simulink model "AGTF30SysDyn_PExPIn"  (R2023b)
settings: Solver=ode4  StartTime=0.0  StopTime=MWS.In.tend  FixedStep=MWS.In.Ts  RelTol=1e-3  EnableMultiTasking=on
model workspace: external: MAT-File (data not in the file)
values from neighbouring files (symbols this model uses):
  MWS = setup_initialize(MWS,startPt,SSsolverSP)    [Setup_Simulation.m]    (also in run_AGTF30e_script.m = Setup_Simulation(inputMethod,MWS.In,filename,Mdl,SSsolverSP))
undefined symbols (not defined in the file or in its folder): DiscIntNeverNeededParam
libraries: simulink x32, Lib_Solve_ModelSource_TMATS x28, Lib_EMTAT x27, Lib_Cntrl_FirstOrderSensor_TMATS x19, Lib_Cntrl_FirstOrderActuator_TMATS x2, Lib_Cntrl_LimitSelect_TMATS x2, Lib_Solve_OuterLoopIntegrator_TMATS x2, Lib_Cntrl_CorrectedSpeed_TMATS x1, Lib_Solve_IterNRSolverJC_TMATS x1, slpidlib x1
(part 3 of 8)

== system AGTF30SysDyn_PExPIn/Control System/Electric Machine Controllers/TEEM Power ==
  k_N1cErrN : Inport
  f_N1cErrN : Inport  Port=2
  Prelookup : Inport  Port=3
  Bus Selector1 : BusSelector  OutputSignals=k_Alt,f_Alt
  Constant : Constant  Value=MWS.In.Options.TEEM
  Constant1 : Constant  Value=0
  PwrExAccel Interpolation Using Prelookup : Interpolation_n-D  Table=MWS.Cntrl.TEEM.PwrExAccel.Pwr_array  InternalRulePriority=Speed
  PwrInAccel Interpolation Using Prelookup : Interpolation_n-D  Table=MWS.Cntrl.TEEM.PwrInAccel.Pwr_array  InternalRulePriority=Speed
  PwrXDecel Interpolation Using Prelookup : Interpolation_n-D  Table=MWS.Cntrl.TEEM.PwrXDecel.Pwr_array  InternalRulePriority=Speed
  Switch : Switch  Criteria=u2 > Threshold  SaturateOnIntegerOverflow=off  InputSameDT=off
  Switch1 : Switch  Criteria=u2 > Threshold  SaturateOnIntegerOverflow=off  InputSameDT=off
  Switch2 : Switch  Criteria=u2 > Threshold  SaturateOnIntegerOverflow=off  InputSameDT=off
  PwrInAccel_TEEM : Outport
  PwrExAccel_TEEM : Outport  Port=2
  PwrXDecel_TEEM : Outport  Port=3
  wires:
  Prelookup/1 -> Bus Selector1/1
  PwrInAccel Interpolation Using Prelookup/1 -> Switch/1  "PwrInAccel_TEEM"
  Bus Selector1/2 -> PwrExAccel Interpolation Using Prelookup/4, PwrInAccel Interpolation Using Prelookup/4, PwrXDecel Interpolation Using Prelookup/4  "<f_Alt>"
  k_N1cErrN/1 -> PwrExAccel Interpolation Using Prelookup/1, PwrInAccel Interpolation Using Prelookup/1, PwrXDecel Interpolation Using Prelookup/1
  PwrXDecel Interpolation Using Prelookup/1 -> Switch1/1  "PwrXDecel_TEEM"
  f_N1cErrN/1 -> PwrExAccel Interpolation Using Prelookup/2, PwrInAccel Interpolation Using Prelookup/2, PwrXDecel Interpolation Using Prelookup/2
  Bus Selector1/1 -> PwrExAccel Interpolation Using Prelookup/3, PwrInAccel Interpolation Using Prelookup/3, PwrXDecel Interpolation Using Prelookup/3  "<k_Alt>"
  Constant/1 -> Switch2/2, Switch1/2, Switch/2
  Switch/1 -> PwrInAccel_TEEM/1
  Switch1/1 -> PwrXDecel_TEEM/1
  PwrExAccel Interpolation Using Prelookup/1 -> Switch2/1  "PwrExAccel_TEEM"
  Constant1/1 -> Switch1/3, Switch2/3, Switch/3
  Switch2/1 -> PwrExAccel_TEEM/1

== system AGTF30SysDyn_PExPIn/Control System/Scheduling/MaxMin Fuel Flow Calc ==
  k_Alt : Inport
  f_Alt : Inport  Port=2
  k_MN : Inport  Port=3
  f_MN : Inport  Port=4
  k_PwrInLPMx : Inport  Port=5
  f_PwrInLPMx : Inport  Port=6
  k_PwrInLPMn : Inport  Port=7
  f_PwrInLPMn : Inport  Port=8
  k_PwrInHPMx : Inport  Port=9
  f_PwrInHPMx : Inport  Port=10
  k_PwrInHPMn : Inport  Port=11
  f_PwrInHPMn : Inport  Port=12
  Wfmax Interpolation Using Prelookup : Interpolation_n-D  NumberOfTableDimensions=4  Table=MWS.Cntrl.Sched.WfMax.WfMax_array  InternalRulePriority=Speed
      settings: InputPortMap=u0,u1,u2,u3,u4,u5,u6,u7
  Wfmin Interpolation Using Prelookup : Interpolation_n-D  NumberOfTableDimensions=4  Table=MWS.Cntrl.Sched.WfMin.WfMin_array  InternalRulePriority=Speed
      settings: InputPortMap=u0,u1,u2,u3,u4,u5,u6,u7
  Wfmin : Outport  VectorParamsAs1DForOutWhenUnconnected=off
  Wfmax : Outport  Port=2  VectorParamsAs1DForOutWhenUnconnected=off
  wires:
  f_PwrInLPMn/1 -> Wfmin Interpolation Using Prelookup/6
  k_PwrInLPMn/1 -> Wfmin Interpolation Using Prelookup/5
  f_PwrInLPMx/1 -> Wfmax Interpolation Using Prelookup/6
  k_PwrInLPMx/1 -> Wfmax Interpolation Using Prelookup/5
  f_MN/1 -> Wfmax Interpolation Using Prelookup/4, Wfmin Interpolation Using Prelookup/4
  k_MN/1 -> Wfmax Interpolation Using Prelookup/3, Wfmin Interpolation Using Prelookup/3
  f_Alt/1 -> Wfmax Interpolation Using Prelookup/2, Wfmin Interpolation Using Prelookup/2
  k_Alt/1 -> Wfmax Interpolation Using Prelookup/1, Wfmin Interpolation Using Prelookup/1
  Wfmin Interpolation Using Prelookup/1 -> Wfmin/1
  Wfmax Interpolation Using Prelookup/1 -> Wfmax/1
  k_PwrInHPMx/1 -> Wfmax Interpolation Using Prelookup/7
  f_PwrInHPMx/1 -> Wfmax Interpolation Using Prelookup/8
  k_PwrInHPMn/1 -> Wfmin Interpolation Using Prelookup/7
  f_PwrInHPMn/1 -> Wfmin Interpolation Using Prelookup/8

== system AGTF30SysDyn_PExPIn/Control System/Scheduling/Power Level Lookup Determination ==
  k_Alt : Inport
  f_Alt : Inport  Port=2
  k_MN : Inport  Port=3
  f_MN : Inport  Port=4
  k_PwrInLPMn : Inport  Port=5
  f_PwrInLPMx : Inport  Port=6
  k_PwrInHPMn : Inport  Port=7
  f_PwrInHPMx : Inport  Port=8
  FnTarget : Inport  Port=9
  N1c : Inport  Port=10
  Constant1 : Constant  Value=MWS.Cntrl.SPSched.PL_vec
  Constant35 : Constant  Value=[[0:1:length(MWS.Cntrl.SPSched.PL_vec)-2],length(MWS.Cntrl.SPSched.PL_vec)-2]
  Constant36 : Constant  Value=[zeros(1,length(MWS.Cntrl.SPSched.PL_vec)-1),1]
  Fn Interpolation Using Prelookup : Interpolation_n-D  NumberOfTableDimensions=5  Table=MWS.Cntrl.Sched.Fn.Fn_array  InternalRulePriority=Speed
      settings: InputPortMap=u0,u1,u2,u3,u4,u5,u6,u7,u8,u9
  Fn Lookup Table Dynamic : simulink/Lookup Tables/Lookup Table Dynamic  LookUpMeth=Interpolation-Use End Values  OutDataType=fixdt('double')  OutScaling=[]  OutputDataTypeScalingMode=Specify via dialog  OutDataTypeStr=double  DoSatur=off
  N1c Interpolation Using Prelookup1 : Interpolation_n-D  NumberOfTableDimensions=5  Table=MWS.Cntrl.WfCntrl.Sched.N1cSP.N1cSP_array  InternalRulePriority=Speed
      settings: InputPortMap=u0,u1,u2,u3,u4,u5,u6,u7,u8,u9
  N1c Lookup Table Dynamic : simulink/Lookup Tables/Lookup Table Dynamic  LookUpMeth=Interpolation-Use End Values  OutDataType=fixdt('double')  OutScaling=[]  OutputDataTypeScalingMode=Specify via dialog  OutDataTypeStr=double  DoSatur=off
  PL Prelookup1 : PreLookup  BreakpointsData=MWS.Cntrl.SPSched.PL_vec  IndexSearchMethod=Linear search  BeginIndexSearchUsingPreviousIndexResult=on  ExtrapMethod=Linear
  PL Targ Prelookup : PreLookup  BreakpointsData=MWS.Cntrl.SPSched.PL_vec  IndexSearchMethod=Linear search  BeginIndexSearchUsingPreviousIndexResult=on  ExtrapMethod=Linear
  k_PL_Targ : Outport
  f_PL_Targ : Outport  Port=2
  k_PL : Outport  Port=3
  f_PL : Outport  Port=4
  wires:
  f_PwrInHPMx/1 -> N1c Interpolation Using Prelookup1/10, Fn Interpolation Using Prelookup/10
  f_PwrInLPMx/1 -> N1c Interpolation Using Prelookup1/8, Fn Interpolation Using Prelookup/8
  k_PwrInHPMn/1 -> N1c Interpolation Using Prelookup1/9, Fn Interpolation Using Prelookup/9
  k_Alt/1 -> N1c Interpolation Using Prelookup1/3, Fn Interpolation Using Prelookup/3
  f_MN/1 -> N1c Interpolation Using Prelookup1/6, Fn Interpolation Using Prelookup/6
  k_MN/1 -> N1c Interpolation Using Prelookup1/5, Fn Interpolation Using Prelookup/5
  Constant35/1 -> N1c Interpolation Using Prelookup1/1, Fn Interpolation Using Prelookup/1
  f_Alt/1 -> N1c Interpolation Using Prelookup1/4, Fn Interpolation Using Prelookup/4
  k_PwrInLPMn/1 -> N1c Interpolation Using Prelookup1/7, Fn Interpolation Using Prelookup/7
  Constant36/1 -> N1c Interpolation Using Prelookup1/2, Fn Interpolation Using Prelookup/2
  Fn Interpolation Using Prelookup/1 -> [FnVec]
  FnTarget/1 -> Fn Lookup Table Dynamic/1
  [FnVec] -> Fn Lookup Table Dynamic/2
  Constant1/1 -> N1c Lookup Table Dynamic/3, Fn Lookup Table Dynamic/3
  Fn Lookup Table Dynamic/1 -> PL Targ Prelookup/1  "PL"
  PL Targ Prelookup/2 -> f_PL_Targ/1  "f_PL_Fn"
  PL Targ Prelookup/1 -> k_PL_Targ/1  "k_PL_Fn"
  N1c Lookup Table Dynamic/1 -> PL Prelookup1/1  "PL"
  PL Prelookup1/2 -> f_PL/1  "f_PL_Fn"
  PL Prelookup1/1 -> k_PL/1  "k_PL_Fn"
  [N1cVec] -> N1c Lookup Table Dynamic/2
  N1c Interpolation Using Prelookup1/1 -> [N1cVec]
  N1c/1 -> N1c Lookup Table Dynamic/1

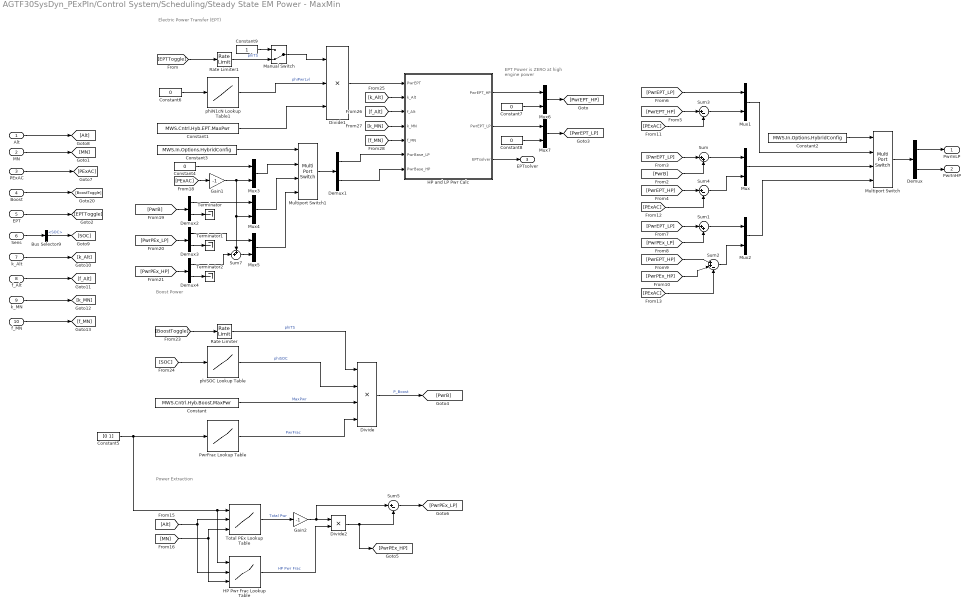
== system AGTF30SysDyn_PExPIn/Control System/Scheduling/Steady State EM Power - MaxMin ==
  note: EPT Power is ZERO at high engine power
  note: Electric Power Transfer (EPT)
  note: Boost Power
  note: Power Extraction
  Alt : Inport
  MN : Inport  Port=2
  PExAC : Inport  Port=3
  Boost : Inport  Port=4
  EPT : Inport  Port=5
  Sens : Inport  Port=6
  k_Alt : Inport  Port=7
  f_Alt : Inport  Port=8
  k_MN : Inport  Port=9
  f_MN : Inport  Port=10
  Bus Selector9 : BusSelector  OutputSignals=SOC
  Constant : Constant  Value=MWS.Cntrl.Hyb.Boost.MaxPwr
  Constant1 : Constant  Value=MWS.Cntrl.Hyb.EPT.MaxPwr
  Constant2 : Constant  Value=MWS.In.Options.HybridConfig
  Constant3 : Constant  Value=MWS.In.Options.HybridConfig
  Constant{4,6..8} (4 alike) : Constant  Value=0
  Constant5 : Constant  Value=[0 1]
  Constant9 : Constant
  Demux{,1..4} (5 alike) : Demux  Outputs=2
  Divide : Product  Inputs=****
  Divide1 : Product  Inputs=***
  Divide2 : Product  Inputs=**
  Gain1 : Gain  Gain=-1
  Gain2 : Gain  Gain=-1
  HP Pwr Frac Lookup Table : Lookup_n-D  NumberOfTableDimensions=3  BreakpointsForDimension1=MWS.Cntrl.Hyb.PEx.PwrSplitSched.NcFanN_vec  BreakpointsForDimension2=MWS.Cntrl.Hyb.PEx.PwrSplitSched.Alt_vec  BreakpointsForDimension3=MWS.Cntrl.Hyb.PEx.PwrSplitSched.MN_vec  Table=MWS.Cntrl.Hyb.PEx.PwrSplitSched.PwrFracHP_array  InternalRulePriority=Speed  RndMeth=Simplest
      settings: InputPortMap=u0,u1,u2
  HP and LP Pwr Calc : Subsystem
  Manual Switch : ManualSwitch  CurrentSetting=0
  Multiport Switch : MultiPortSwitch  SaturateOnIntegerOverflow=off  InputSameDT=off
  Multiport Switch1 : MultiPortSwitch  SaturateOnIntegerOverflow=off  InputSameDT=off
  Mux{,1..7} (8 alike) : Mux  Inputs=2
  PwrFrac Lookup Table : Lookup_n-D  NumberOfTableDimensions=1  BreakpointsForDimension1=MWS.Cntrl.Hyb.Boost.PwrFracSched.NcFanN_vec  BreakpointsForDimension2=MWS.Cntrl.PHpwr.Sched.MN_vec  Table=MWS.Cntrl.Hyb.Boost.PwrFracSched.PwrFrac_vec  InternalRulePriority=Speed  RndMeth=Simplest
  Rate Limiter : RateLimiter  RisingSlewLimit=MWS.Cntrl.Hyb.Boost.RL  FallingSlewLimit=-MWS.Cntrl.Hyb.Boost.RL  SampleTimeMode=inherited
  Rate Limiter1 : RateLimiter  RisingSlewLimit=MWS.Cntrl.Hyb.EPT.RL  FallingSlewLimit=-MWS.Cntrl.Hyb.EPT.RL  SampleTimeMode=inherited
  Sum : Sum  Inputs=|++
  Sum1 : Sum  Inputs=|++
  Sum2 : Sum  Inputs=|++-
  Sum3 : Sum  Inputs=|+-
  Sum4 : Sum  Inputs=|+-
  Sum5 : Sum  Inputs=|+-
  Sum7 : Sum  Inputs=++|
  Terminator : Terminator
  Terminator1 : Terminator
  Terminator2 : Terminator
  Total PEx Lookup Table : Lookup_n-D  NumberOfTableDimensions=3  BreakpointsForDimension1=MWS.Cntrl.Hyb.PEx.PExSched.NcFanN_vec  BreakpointsForDimension2=MWS.Cntrl.Hyb.PEx.PExSched.Alt_vec  BreakpointsForDimension3=MWS.Cntrl.Hyb.PEx.PExSched.MN_vec  Table=MWS.Cntrl.Hyb.PEx.PExSched.Pwr_array  InternalRulePriority=Speed  RndMeth=Simplest
      settings: InputPortMap=u0,u1,u2
  phiN1cN Lookup Table1 : Lookup_n-D  NumberOfTableDimensions=1  BreakpointsForDimension1=MWS.Cntrl.Hyb.EPT.Sched.N1cN_vec  BreakpointsForDimension2=MWS.Cntrl.PHpwr.Sched.MN_vec  Table=MWS.Cntrl.Hyb.EPT.Sched.phiPwrLvl_vec  InternalRulePriority=Speed  RndMeth=Simplest
  phiSOC Lookup Table : Lookup_n-D  NumberOfTableDimensions=1  BreakpointsForDimension1=MWS.Cntrl.Hyb.Boost.phiSOCSched.SOC_vec  BreakpointsForDimension2=MWS.Cntrl.PHpwr.Sched.MN_vec  Table=MWS.Cntrl.Hyb.Boost.phiSOCSched.phiSOC_vec  InternalRulePriority=Speed  RndMeth=Simplest
  PwrInLP : Outport
  PwrInHP : Outport  Port=2
  EPTsolver : Outport  Port=3
  wires:
  Constant/1 -> Divide/3  "MaxPwr"
  MN/1 -> [MN]
  [SOC] -> phiSOC Lookup Table/1
  phiSOC Lookup Table/1 -> Divide/2  "phiSOC"
  [BoostToggle] -> Rate Limiter/1
  Alt/1 -> [Alt]
  PwrFrac Lookup Table/1 -> Divide/4  "PwrFrac"
  Sens/1 -> Bus Selector9/1
  Rate Limiter/1 -> Divide/1  "phiTS"
  Boost/1 -> [BoostToggle]
  Divide/1 -> [PwrB]  "P_Boost"
  [EPTToggle] -> Rate Limiter1/1
  Constant6/1 -> phiN1cN Lookup Table1/1
  phiN1cN Lookup Table1/1 -> Divide1/2  "phiPwrLvl"
  Rate Limiter1/1 -> Manual Switch/2  "phiTS"
  [PwrEPT_LP] -> Sum/1
  [PwrB] -> Sum/2
  [PwrEPT_LP] -> Mux1/1
  Sum/1 -> Mux/1
  [PwrEPT_HP] -> Sum4/1
  [PwrEPT_LP] -> Sum1/1
  [PwrPEx_LP] -> Sum1/2
  [PwrEPT_HP] -> Sum2/1
  [PwrPEx_HP] -> Sum2/2
  Sum2/1 -> Mux2/2
  Sum1/1 -> Mux2/1
  Mux1/1 -> Multiport Switch/2
  Mux/1 -> Multiport Switch/3
  Mux2/1 -> Multiport Switch/4
  Constant2/1 -> Multiport Switch/1
  [PwrEPT_HP] -> Sum3/1
  [PExAC] -> Sum3/2
  Sum3/1 -> Mux1/2
  Multiport Switch/1 -> Demux/1
  Demux/1 -> PwrInLP/1
  [PExAC] -> Sum4/2
  [PExAC] -> Sum2/3
  Sum4/1 -> Mux/2
  Constant5/1 -> HP Pwr Frac Lookup Table/1, Total PEx Lookup Table/1, PwrFrac Lookup Table/1
  [Alt] -> HP Pwr Frac Lookup Table/2, Total PEx Lookup Table/2
  [MN] -> HP Pwr Frac Lookup Table/3, Total PEx Lookup Table/3
  Total PEx Lookup Table/1 -> Gain2/1  "Total Pwr"
  HP Pwr Frac Lookup Table/1 -> Divide2/2  "HP Pwr Frac"
  Divide2/1 -> [PwrPEx_HP], Sum5/2
  Gain2/1 -> Divide2/1, Sum5/1
  Sum5/1 -> [PwrPEx_LP]
  EPT/1 -> [EPTToggle]
  PExAC/1 -> [PExAC]
  Constant1/1 -> Divide1/3
  Bus Selector9/1 -> [SOC]  "<SOC>"
  Constant3/1 -> Multiport Switch1/1
  Constant4/1 -> Mux3/1
  [PExAC] -> Gain1/1
  Mux3/1 -> Multiport Switch1/2
  Gain1/1 -> Mux3/2, Mux4/2, Sum7/1
  Sum7/1 -> Mux5/2
  Mux4/1 -> Multiport Switch1/3
  Mux5/1 -> Multiport Switch1/4
  Multiport Switch1/1 -> Demux1/1
  Demux1/1 -> HP and LP Pwr Calc/6(PwrBase_LP)
  Demux1/2 -> HP and LP Pwr Calc/7(PwrBase_HP)
  k_Alt/1 -> [k_Alt]
  f_Alt/1 -> [f_Alt]
  k_MN/1 -> [k_MN]
  f_MN/1 -> [f_MN]
  [f_Alt] -> HP and LP Pwr Calc/3(f_Alt)
  [k_MN] -> HP and LP Pwr Calc/4(k_MN)
  [f_MN] -> HP and LP Pwr Calc/5(f_MN)
  [k_Alt] -> HP and LP Pwr Calc/2(k_Alt)
  Divide1/1 -> HP and LP Pwr Calc/1(PwrEPT)
  HP and LP Pwr Calc/3(EPTsolver) -> EPTsolver/1
  Mux6/1 -> [PwrEPT_HP]
  Mux7/1 -> [PwrEPT_LP]
  HP and LP Pwr Calc/1(PwrEPT_HP) -> Mux6/1
  HP and LP Pwr Calc/2(PwrEPT_LP) -> Mux7/1
  Constant7/1 -> Mux6/2
  Constant8/1 -> Mux7/2
  Demux2/2 -> Terminator/1
  [PwrB] -> Demux2/1
  Demux2/1 -> Mux4/1
  [PwrPEx_LP] -> Demux3/1
  [PwrPEx_HP] -> Demux4/1
  Demux3/2 -> Terminator1/1
  Demux4/2 -> Terminator2/1
  Demux4/1 -> Sum7/2
  Demux3/1 -> Mux5/1
  Constant9/1 -> Manual Switch/1
  Manual Switch/1 -> Divide1/1
  Demux/2 -> PwrInHP/1

== system AGTF30SysDyn_PExPIn/Control System/Wf Controller/Controller ==
  Prelookup : Inport
  Alt : Inport  Port=2
  MN : Inport  Port=3
  N1c : Inport  Port=4
  N1 : Inport  Port=5
  N3 : Inport  Port=6
  Ps3 : Inport  Port=7
  T3 : Inport  Port=8
  T4 : Inport  Port=9
  T45 : Inport  Port=10
  NcFanManEn : Inport  Port=11
  NcFanMan : Inport  Port=12
  Wfmin : Inport  Port=13
  Wfmax : Inport  Port=14
  phiEPT : Inport  Port=15
  phiBoost : Inport  Port=16
  N1cN : Inport  Port=17
  Bus Creator : BusCreator  Inputs=2
  Mux1 : Mux  Inputs=7
  Mux2 : Mux  Inputs=3
  N1cSP Limit Controllers : Subsystem
  N1cSP Limit Select : Subsystem
  Nominal Controller : Subsystem
  Nominal Set-Point Determination : Subsystem
  Set-Points : Subsystem
  Wf Limit Controllers : Subsystem
  Wf Limit Select : Subsystem
  Wfdmd : Outport  VectorParamsAs1DForOutWhenUnconnected=off
  RegNum : Outport  Port=2  VectorParamsAs1DForOutWhenUnconnected=off
  SPs : Outport  Port=3  VectorParamsAs1DForOutWhenUnconnected=off
  N1cErr : Outport  Port=4  VectorParamsAs1DForOutWhenUnconnected=off
  wires:
  N1c/1 -> Nominal Controller/5(N1c)
  Prelookup/1 -> [Prelookup], N1cSP Limit Controllers/1(Prelookup), Nominal Set-Point Determination/1(Prelookup)
  N1cSP Limit Select/1(N1cSPdmd) -> Nominal Controller/4(N1cSP), N1cSP Limit Controllers/8(N1cCmd)
  T4/1 -> N1cSP Limit Controllers/6(T4)
  N3/1 -> N1cSP Limit Controllers/3(N3)
  Ps3/1 -> Wf Limit Controllers/9(ps3), N1cSP Limit Controllers/4(Ps3)
  T3/1 -> N1cSP Limit Controllers/5(T3)
  Nominal Set-Point Determination/1(N1cSP) -> Set-Points/1(Nominal SP), N1cSP Limit Select/1(N1cSPReq)
  N1cSP Limit Controllers/8(SPs) -> Set-Points/2(N1cSP Limit SPs)
  Set-Points/1(SPs) -> SPs/1
  N1/1 -> N1cSP Limit Controllers/2(N1)
  N1cSP Limit Controllers/7(N1cSP Ps3 Min) -> Mux1/7
  N1cSP Limit Controllers/5(N1cSP N3 Max) -> Mux1/5
  N1cSP Limit Controllers/4(N1cSP N1 Max) -> Mux1/4
  N1cSP Limit Controllers/6(N1cSP Ps3 Max) -> Mux1/6
  N1cSP Limit Controllers/2(N1cSP T4 Max) -> Mux1/2
  NcFanManEn/1 -> Nominal Controller/2(N1cManEn)
  N1cSP Limit Controllers/1(N1cSP T3 Max) -> Mux1/1
  [Prelookup] -> Nominal Controller/1(Prelookup)
  Nominal Controller/1(Wfdmd) -> Wf Limit Select/1(WfReq)
  Wf Limit Select/1(Wfdmd) -> Nominal Controller/6(Wfcmd), Wf Limit Controllers/5(Wfcmd), Wfdmd/1
  Wfmin/1 -> Wf Limit Controllers/3(Wfmin)
  Wfmax/1 -> Wf Limit Controllers/4(Wfmax)
  Wf Limit Controllers/1(Wf Accel) -> Mux2/1
  Wf Limit Controllers/2(Wf Decel) -> Mux2/2
  Wf Limit Controllers/3(Wf Min) -> Mux2/3
  Mux2/1 -> Wf Limit Select/2(Limits)
  Wf Limit Controllers/4(SPs) -> Set-Points/3(Wf Limit SPs)
  Alt/1 -> Wf Limit Controllers/1(Alt)
  T45/1 -> N1cSP Limit Controllers/7(T45)
  N1cSP Limit Controllers/3(N1cSP T45 Max) -> Mux1/3
  NcFanMan/1 -> Nominal Controller/3(N1cMan)
  Bus Creator/1 -> RegNum/1
  N1cSP Limit Select/2(RegNum) -> Wf Limit Controllers/10(RegNum), Bus Creator/1  "N1cSP"
  Wf Limit Select/2(RegNum) -> Bus Creator/2  "Wf"
  Nominal Controller/2(N1cErr) -> N1cErr/1
  Mux1/1 -> N1cSP Limit Select/2(Limits)
  MN/1 -> Wf Limit Controllers/2(MN)
  phiEPT/1 -> Wf Limit Controllers/6(phiEPT)
  phiBoost/1 -> Wf Limit Controllers/7(phiBoost)
  N1cN/1 -> Wf Limit Controllers/8(N1cN)

== system AGTF30SysDyn_PExPIn/Control System/Wf Controller/Corrected Speed Calc ==
  N : Inport
  T : Inport  Port=2
  Divide : Product  Inputs=*/
  Gain : Gain  Gain=1/518.67
  Sqrt : Sqrt
  Nc : Outport  VectorParamsAs1DForOutWhenUnconnected=off
  wires:
  Sqrt/1 -> Divide/2
  N/1 -> Divide/1
  T/1 -> Gain/1
  Gain/1 -> Sqrt/1
  Divide/1 -> Nc/1

== system AGTF30SysDyn_PExPIn/EngineSystem/EngineDW/Subsystem ==
  SysIn : Inport
  N : Inport  Port=2
  Bus Selector4 : BusSelector  OutputSignals=CntrlInp.ManualOp.PwrInLPNomMan,CntrlInp.ManualOp.PwrInLPNomManEn,CntrlInp.ManualOp.PwrInLPOffNomMan,CntrlInp.ManualOp.PwrInLPOffNomManEn,CntrlInp.ManualOp.PwrInHPNomMan,CntrlInp.ManualOp.PwrInHPNomManEn,CntrlInp.ManualOp.PwrInHPOffNomMan,CntrlInp.ManualOp.PwrInHPOffNomManEn
  Constant{,1..3} (4 alike) : Constant  Value=0
  Demux : Demux  Outputs=2
  Divide : Product  Inputs=*/
  Divide1 : Product  Inputs=/*
  Gain : Gain  Gain=5252.113
  Gain1 : Gain  Gain=5252.113
  Sum : Sum  Inputs=|++
  Sum1 : Sum  Inputs=|++
  Switch{,1..3} (4 alike) : Switch  Criteria=u2 > Threshold  SaturateOnIntegerOverflow=off  InputSameDT=off
  TrqInLP : Outport
  TrqInHP : Outport  Port=2
  wires:
  SysIn/1 -> Bus Selector4/1
  Bus Selector4/1 -> [PwrLPNom]  "<PwrInLPNomMan>"
  Bus Selector4/2 -> [EnPwrLPNom]  "<PwrInLPNomManEn>"
  Bus Selector4/3 -> [PwrLPOffNom]  "<PwrInLPOffNomMan>"
  Bus Selector4/4 -> [EnPwrLPOffNom]  "<PwrInLPOffNomManEn>"
  [EnPwrLPNom] -> Switch/2
  Constant/1 -> Switch/3
  [PwrLPNom] -> Switch/1
  [PwrLPOffNom] -> Switch1/1
  Constant1/1 -> Switch1/3
  [EnPwrLPOffNom] -> Switch1/2
  Switch/1 -> Sum/1
  Switch1/1 -> Sum/2
  Sum/1 -> Divide/1
  Sum1/1 -> Divide1/2
  Switch3/1 -> Sum1/2
  Switch2/1 -> Sum1/1
  [EnPwrHPOffNom] -> Switch3/2
  Constant3/1 -> Switch3/3
  [PwrHPOffNom] -> Switch3/1
  [PwrHPNom] -> Switch2/1
  Constant2/1 -> Switch2/3
  [EnPwrHPNom] -> Switch2/2
  Bus Selector4/5 -> [PwrHPNom]  "<PwrInHPNomMan>"
  Bus Selector4/6 -> [EnPwrHPNom]  "<PwrInHPNomManEn>"
  Bus Selector4/7 -> [PwrHPOffNom]  "<PwrInHPOffNomMan>"
  Bus Selector4/8 -> [EnPwrHPOffNom]  "<PwrInHPOffNomManEn>"
  N/1 -> Demux/1
  Divide/1 -> Gain/1
  Gain/1 -> TrqInLP/1
  Divide1/1 -> Gain1/1
  Gain1/1 -> TrqInHP/1
  Demux/1 -> Divide/2
  Demux/2 -> Divide1/1

== system AGTF30SysDyn_PExPIn/EngineSystem/Power System/Electrical Power System ==
  note: Author: Jackson Steiner (modified by Jonathan Kratz)
      | Updated: 2024-08-06 (modified 2024-09-19)
  NemL [rpm] : Inport
  TrqEML [ft-lb] : Inport  Port=2
  NemH [rpm] : Inport  Port=3
  TrqEMH [ft-lb] : Inport  Port=4
  NemS [rpm] : Inport  Port=5
  TrqEMS [ft-lb] : Inport  Port=6
  NemR [rpm] : Inport  Port=7
  TrqEMR [ft-lb] : Inport  Port=8
  NemC [rpm] : Inport  Port=9
  TrqEMC [ft-lb] : Inport  Port=10
  NemP [rpm] : Inport  Port=11
  TrqEMP [ft-lb] : Inport  Port=12
  Load [hp] : Inport  Port=13
  EM Variant Subsystem : Subsystem  Variant=on
  Energy Storage Subsystem : Subsystem
  Out_LPEMbranch : Outport
  Out_HPEMbranch : Outport  Port=2
  Out_SEMbranch : Outport  Port=3
  Out_REMbranch : Outport  Port=4
  Out_CEMbranch : Outport  Port=5
  Out_PEMbranch : Outport  Port=6
  Out_SupplySys : Outport  Port=7  OutDataTypeStr=Bus: SuppSys_Bus
  SoC [%] : Outport  Port=8
  wires:
  EM Variant Subsystem/5(Out_REMbranch) -> Out_REMbranch/1
  EM Variant Subsystem/6(Out_CEMbranch) -> Out_CEMbranch/1
  [V_DC_Out] -> EM Variant Subsystem/1(Vs [V])
  EM Variant Subsystem/7(Out_PEMbranch) -> Out_PEMbranch/1
  EM Variant Subsystem/4(Out_SEMbranch) -> Out_SEMbranch/1
  EM Variant Subsystem/2(Out_LPEMbranch) -> Out_LPEMbranch/1
  EM Variant Subsystem/3(Out_HPEMbranch) -> Out_HPEMbranch/1
  TrqEML [ft-lb]/1 -> EM Variant Subsystem/3(TrqEML [ft-lb])
  NemL [rpm]/1 -> EM Variant Subsystem/2(NemL [rpm])
  NemH [rpm]/1 -> EM Variant Subsystem/4(NemH [rpm])
  TrqEMP [ft-lb]/1 -> EM Variant Subsystem/13(TrqEMP [ft-lb])
  NemS [rpm]/1 -> EM Variant Subsystem/6(NemS [rpm])
  TrqEMS [ft-lb]/1 -> EM Variant Subsystem/7(TrqEMS [ft-lb])
  NemR [rpm]/1 -> EM Variant Subsystem/8(NemR [rpm])
  TrqEMH [ft-lb]/1 -> EM Variant Subsystem/5(TrqEMH [ft-lb])
  NemC [rpm]/1 -> EM Variant Subsystem/10(NemC [rpm])
  TrqEMR [ft-lb]/1 -> EM Variant Subsystem/9(TrqEMR [ft-lb])
  NemP [rpm]/1 -> EM Variant Subsystem/12(NemP [rpm])
  TrqEMC [ft-lb]/1 -> EM Variant Subsystem/11(TrqEMC [ft-lb])
  Energy Storage Subsystem/3(SoC [%]) -> SoC [%]/1
  Energy Storage Subsystem/2(Out_SupplySys) -> Out_SupplySys/1
  Energy Storage Subsystem/1(V_DC_Out [V]) -> [V_DC_Out]
  EM Variant Subsystem/1(Io [A]) -> Energy Storage Subsystem/1(I_2 [A])
  Load [hp]/1 -> Energy Storage Subsystem/2(Load [hp])

== system AGTF30SysDyn_PExPIn/Control System/Electric Machine Controllers/EM Controllers/DEM Control ==
  PwrInLPEMNomMan : Inport
  PwrInLPEMNomManEn : Inport  Port=2
  PwrInLPEMOffNomMan : Inport  Port=3
  PwrInLPEMOffNomManEn : Inport  Port=4
  PwrInHPEMNomMan : Inport  Port=5
  PwrInHPEMNomManEn : Inport  Port=6
  PwrInHPEMOffNomMan : Inport  Port=7
  PwrInHPEMOffNomManEn : Inport  Port=8
  PwrInLP_Base : Inport  Port=9
  PwrInHP_Base : Inport  Port=10
  NemL : Inport  Port=11
  NemH : Inport  Port=12
  PwrEPT : Inport  Port=13
  PwrInAccel_TEEM : Inport  Port=14
  PwrExAccel_TEEM : Inport  Port=15
  PwrXDecel_TEEM : Inport  Port=16
  PwrCharge : Inport  Port=17
  PExAC : Inport  Port=18
  PwrSys : Inport  Port=19
  Constant : Constant  Value=0
  DEM EM Controllers : Subsystem
  PwrEML : Outport
  TrqEML : Outport  Port=2
  PwrEMH : Outport  Port=3
  TrqEMH : Outport  Port=4
  PwrEMS : Outport  Port=5
  TrqEMS : Outport  Port=6
  PwrEMR : Outport  Port=7
  TrqEMR : Outport  Port=8
  PwrEMC : Outport  Port=9
  TrqEMC : Outport  Port=10
  PwrEMP : Outport  Port=11
  TrqEMP : Outport  Port=12
  PwrLoad : Outport  Port=13
  wires:
  PwrInLPEMNomMan/1 -> DEM EM Controllers/1(PwrInLPEMNomMan)
  PwrInLPEMNomManEn/1 -> DEM EM Controllers/2(PwrInLPEMNomManEn)
  PwrInLPEMOffNomMan/1 -> DEM EM Controllers/3(PwrInLPEMOffNomMan)
  PwrInLPEMOffNomManEn/1 -> DEM EM Controllers/4(PwrInLPEMOffNomManEn)
  PwrInHPEMNomMan/1 -> DEM EM Controllers/5(PwrInHPEMNomMan)
  PwrInHPEMNomManEn/1 -> DEM EM Controllers/6(PwrInHPEMNomManEn)
  PwrInHPEMOffNomMan/1 -> DEM EM Controllers/7(PwrInHPEMOffNomMan)
  PwrInHPEMOffNomManEn/1 -> DEM EM Controllers/8(PwrInHPEMOffNomManEn)
  PwrInLP_Base/1 -> DEM EM Controllers/9(PwrInLP_Base)
  PwrInHP_Base/1 -> DEM EM Controllers/10(PwrInHP_Base)
  NemL/1 -> DEM EM Controllers/11(NemL)
  NemH/1 -> DEM EM Controllers/12(NemH)
  PwrEPT/1 -> DEM EM Controllers/13(PwrEPT)
  PwrInAccel_TEEM/1 -> DEM EM Controllers/14(PwrInAccel_TEEM)
  PwrExAccel_TEEM/1 -> DEM EM Controllers/15(PwrExAccel_TEEM)
  PwrXDecel_TEEM/1 -> DEM EM Controllers/16(PwrXDecel_TEEM)
  PwrCharge/1 -> DEM EM Controllers/17(PwrCharge)
  PExAC/1 -> DEM EM Controllers/18(PExAC)
  PwrSys/1 -> DEM EM Controllers/19(PwrSys)
  DEM EM Controllers/5(PwrLoad) -> PwrLoad/1
  DEM EM Controllers/4(TrqEMH) -> TrqEMH/1
  DEM EM Controllers/3(TrqEML) -> TrqEML/1
  DEM EM Controllers/2(PwrEMH) -> PwrEMH/1
  DEM EM Controllers/1(PwrEML) -> PwrEML/1
  Constant/1 -> TrqEMP/1, PwrEMP/1, TrqEMC/1, PwrEMC/1, TrqEMR/1, PwrEMR/1, TrqEMS/1, PwrEMS/1

== system AGTF30SysDyn_PExPIn/Control System/Electric Machine Controllers/EM Controllers/PGB EM Control ==
  PwrInSEMNomMan : Inport
  PwrInSEMNomManEn : Inport  Port=2
  PwrInSEMOffNomMan : Inport  Port=3
  PwrInSEMOffNomManEn : Inport  Port=4
  PwrInREMNomMan : Inport  Port=5
  PwrInREMNomManEn : Inport  Port=6
  PwrInREMOffNomMan : Inport  Port=7
  PwrInREMOffNomManEn : Inport  Port=8
  PwrInCEMNomMan : Inport  Port=9
  PwrInCEMNomManEn : Inport  Port=10
  PwrInCEMOffNomMan : Inport  Port=11
  PwrInCEMOffNomManEn : Inport  Port=12
  PwrInPEMNomMan : Inport  Port=13
  PwrInPEMNomManEn : Inport  Port=14
  PwrInPEMOffNomMan : Inport  Port=15
  PwrInPEMOffNomManEn : Inport  Port=16
  PwrInLP_Base : Inport  Port=17
  PwrInHP_Base : Inport  Port=18
  NemS : Inport  Port=19
  NemR : Inport  Port=20
  NemC : Inport  Port=21
  NemP : Inport  Port=22
  PwrEPT : Inport  Port=23
  PwrInAccel_TEEM : Inport  Port=24
  PwrExAccel_TEEM : Inport  Port=25
  PwrXDecel_TEEM : Inport  Port=26
  PwrCharge : Inport  Port=27
  N1cErrN : Inport  Port=28
  PExAC : Inport  Port=29
  PwrSys : Inport  Port=30
  Constant : Constant  Value=0
  VEATE EM Controllers : Subsystem
  PwrEMS : Outport
  TrqEMS : Outport  Port=2
  PwrEMR : Outport  Port=3
  TrqEMR : Outport  Port=4
  PwrEMC : Outport  Port=5
  TrqEMC : Outport  Port=6
  PwrEMP : Outport  Port=7
  TrqEMP : Outport  Port=8
  PwrEML : Outport  Port=9
  PwrEMH : Outport  Port=10
  TrqEML : Outport  Port=11
  TrqEMH : Outport  Port=12
  PwrLoad : Outport  Port=13
  wires:
  PwrSys/1 -> VEATE EM Controllers/30(PwrSys)
  PExAC/1 -> VEATE EM Controllers/29(PExAC)
  N1cErrN/1 -> VEATE EM Controllers/28(N1cErrN)
  PwrCharge/1 -> VEATE EM Controllers/27(PwrCharge)
  PwrXDecel_TEEM/1 -> VEATE EM Controllers/26(PwrXDecel_TEEM)
  PwrExAccel_TEEM/1 -> VEATE EM Controllers/25(PwrExAccel_TEEM)
  PwrInAccel_TEEM/1 -> VEATE EM Controllers/24(PwrInAccel_TEEM)
  PwrEPT/1 -> VEATE EM Controllers/23(PwrEPT)
  NemP/1 -> VEATE EM Controllers/22(NemP)
  NemC/1 -> VEATE EM Controllers/21(NemC)
  NemS/1 -> VEATE EM Controllers/19(NemS)
  NemR/1 -> VEATE EM Controllers/20(NemR)
  PwrInHP_Base/1 -> VEATE EM Controllers/18(PwrInHP_Base)
  VEATE EM Controllers/6(TrqEMC) -> TrqEMC/1
  VEATE EM Controllers/7(PwrEMP) -> PwrEMP/1
  VEATE EM Controllers/8(TrqEMP) -> TrqEMP/1
  VEATE EM Controllers/9(PwrLoad) -> PwrLoad/1
  VEATE EM Controllers/5(PwrEMC) -> PwrEMC/1
  VEATE EM Controllers/4(TrqEMR) -> TrqEMR/1
  VEATE EM Controllers/3(PwrEMR) -> PwrEMR/1
  PwrInLP_Base/1 -> VEATE EM Controllers/17(PwrInLP_Base)
  PwrInPEMOffNomManEn/1 -> VEATE EM Controllers/16(PwrInPEMOffNomManEn)
  PwrInPEMOffNomMan/1 -> VEATE EM Controllers/15(PwrInPEMOffNomMan)
  PwrInPEMNomManEn/1 -> VEATE EM Controllers/14(PwrInPEMNomManEn)
  PwrInPEMNomMan/1 -> VEATE EM Controllers/13(PwrInPEMNomMan)
  PwrInCEMOffNomManEn/1 -> VEATE EM Controllers/12(PwrInCEMOffNomManEn)
  PwrInCEMOffNomMan/1 -> VEATE EM Controllers/11(PwrInCEMOffNomMan)
  PwrInCEMNomManEn/1 -> VEATE EM Controllers/10(PwrInCEMNomManEn)
  PwrInCEMNomMan/1 -> VEATE EM Controllers/9(PwrInCEMNomMan)
  PwrInREMOffNomManEn/1 -> VEATE EM Controllers/8(PwrInREMOffNomManEn)
  PwrInREMOffNomMan/1 -> VEATE EM Controllers/7(PwrInREMOffNomMan)
  VEATE EM Controllers/1(PwrEMS) -> PwrEMS/1
  VEATE EM Controllers/2(TrqEMS) -> TrqEMS/1
  PwrInREMNomManEn/1 -> VEATE EM Controllers/6(PwrInREMNomManEn)
  PwrInREMNomMan/1 -> VEATE EM Controllers/5(PwrInREMNomMan)
  PwrInSEMOffNomManEn/1 -> VEATE EM Controllers/4(PwrInSEMOffNomManEn)
  PwrInSEMOffNomMan/1 -> VEATE EM Controllers/3(PwrInSEMOffNomMan)
  PwrInSEMNomManEn/1 -> VEATE EM Controllers/2(PwrInSEMNomManEn)
  PwrInSEMNomMan/1 -> VEATE EM Controllers/1(PwrInSEMNomMan)
  Constant/1 -> PwrEML/1, TrqEML/1, TrqEMH/1, PwrEMH/1

== system AGTF30SysDyn_PExPIn/Control System/Electric Machine Controllers/SOC Controller/Set Point Controller (PI) ==
  note: PI controller
  note: windup protection
  note: bypass controller and manually set the effector value
  Input_req : Inport
  Input_sensed : Inport  Port=2
  Eff_dmd : Inport  Port=3
  Kp : Inport  Port=4
  Ki : Inport  Port=5
  Man_En : Inport  Port=6
  Eff_Man : Inport  Port=7
  1/sum(Ji)2 : Gain  Gain=WGain_M  SaturateOnIntegerOverflow=on  OutDataTypeStr=Inherit: Same as input  ParamDataTypeStr=Inherit: Same as input
  Add1 : Sum  Inputs=+-
  Constant1 : Constant  Value=PI_IC_M
  Discrete-Time Integrator1 : DiscreteIntegrator  SampleTime=Ts_M  LimitOutput=on  UpperSaturationLimit=MWS.Cntrl.SOCReg.PwrCharge.IntSat  LowerSaturationLimit=-MWS.Cntrl.SOCReg.PwrCharge.IntSat  ICPrevOutput=DiscIntNeverNeededParam  ICPrevScaledInput=DiscIntNeverNeededParam
  Product : Product
  Product1 : Product  Inputs=1
  Product2 : Product
  Product3 : Product  Inputs=1
  Relational Operator : RelationalOperator  Operator===  OutDataTypeStr=boolean  InputSameDT=off
  Sum : Sum  Inputs=|++
  Sum1 : Sum  Inputs=|-+
  Sum2 : Sum  Inputs=|+-
  Sum3 : Sum  Inputs=|++
  Switch : Switch  Criteria=u2 > Threshold  SaturateOnIntegerOverflow=off  InputSameDT=off
  Eff_req : Outport
  Active : Outport  Port=2
  wires:
  Man_En/1 -> Switch/2
  Eff_Man/1 -> Switch/1
  Constant1/1 -> Sum/2
  Sum3/1 -> Sum/1
  Sum/1 -> Switch/3
  Product3/1 -> Product/1
  Product1/1 -> Product2/1
  Kp/1 -> Product1/1
  Relational Operator/1 -> Active/1
  Ki/1 -> Product3/1
  Product/1 -> Discrete-Time Integrator1/1
  Sum2/1 -> Product/2
  1/sum(Ji)2/1 -> Sum2/2
  Sum1/1 -> 1/sum(Ji)2/1
  Eff_dmd/1 -> Relational Operator/2, Sum1/1
  Switch/1 -> Eff_req/1, Sum1/2, Relational Operator/1
  Discrete-Time Integrator1/1 -> Sum3/2
  Input_req/1 -> Add1/1
  Product2/1 -> Sum3/1
  Input_sensed/1 -> Add1/2
  Add1/1 -> Sum2/1, Product2/2

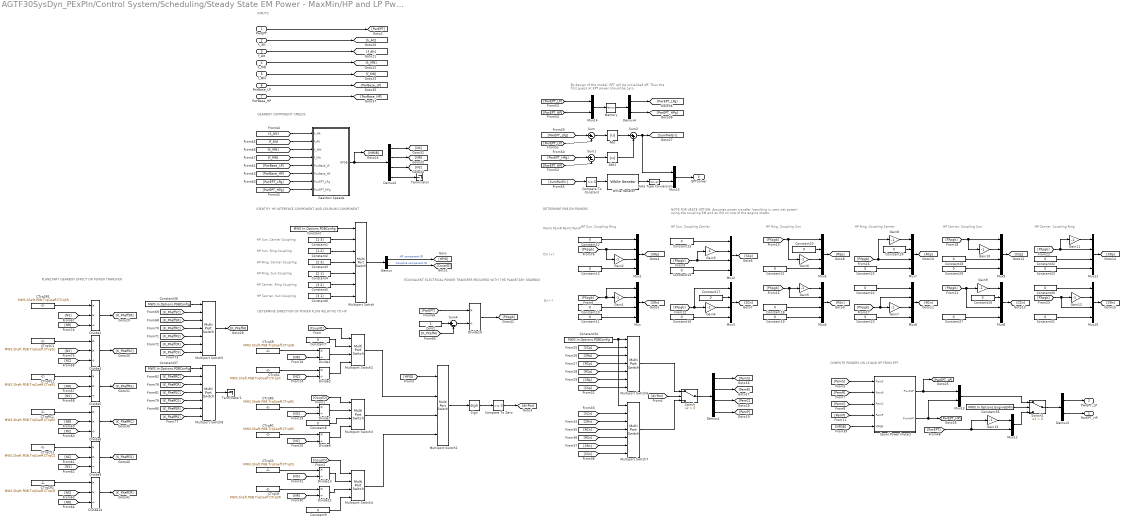
== system AGTF30SysDyn_PExPIn/Control System/Scheduling/Steady State EM Power - MaxMin/HP and LP Pwr Calc ==
  note: By design of the model, EPT will be initialized off. Thus the first guess at EPT power should be zero.
  note: NOTE FOR VEATE OPTION: Assumes power transfer (resulting in zero net power) using the coupling EM and an EM on one of the engine shafts.
  note: Dir (+)
  note: HP Sun, Coupling Ring
  note: PemS
      | PemR
      | PemC
      | PemP
  note: IDENTIFY HP INTERFACE COMPONENT AND COUPLING COMPONENT
  note: HP Sun, Carrier Coupling
  note: HP Sun, Ring Coupling
  note: HP Ring, Carrier Coupling
  note: HP Ring, Sun Coupling
  note: HP Carrier, Ring Coupling
  note: HP Carrier, Sun Coupling
  note: HP Sun, Coupling Carrier
  note: Dir (-)
  note: HP Ring, Coupling Sun
  note: HP Ring, Coupling Carrier
  note: HP Carrier, Coupling Sun
  note: HP Carrier, Coupling Ring
  note: DETERMINE DIRECTION OF POWER FLOW RELATIVE TO HP
  note: DETERMINE PGB EM POWERS
  note: COMPUTE POWERS ON LP AND HP FROM EPT
  note: GEARBOX COMPONENT SPEEDS
  note: INPUTS
  note: PLANETARY GEARBOX EFFECT ON POWER TRANSFER
  note: EQUIVALENT ELECTRICAL POWER TRANSFER REQUIRED WITH THE PLANETARY GEARBOX
  PwrEPT : Inport
  k_Alt : Inport  Port=2
  f_Alt : Inport  Port=3
  k_MN : Inport  Port=4
  f_MN : Inport  Port=5
  PwrBase_LP : Inport  Port=6
  PwrBase_HP : Inport  Port=7
  Abs : Abs  SaturateOnIntegerOverflow=off
  Abs1 : Abs  SaturateOnIntegerOverflow=off
  CTrqCR : Constant  Value=MWS.Shaft.PGB.TrqCoeff.CTrqCR
  CTrqCR1 : Constant  Value=MWS.Shaft.PGB.TrqCoeff.CTrqCR
  CTrqCS : Constant  Value=MWS.Shaft.PGB.TrqCoeff.CTrqCS
  CTrqCS1 : Constant  Value=MWS.Shaft.PGB.TrqCoeff.CTrqCS
  CTrqRC : Constant  Value=MWS.Shaft.PGB.TrqCoeff.CTrqRC
  CTrqRC1 : Constant  Value=MWS.Shaft.PGB.TrqCoeff.CTrqRC
  CTrqRS : Constant  Value=MWS.Shaft.PGB.TrqCoeff.CTrqRS
  CTrqRS1 : Constant  Value=MWS.Shaft.PGB.TrqCoeff.CTrqRS
  CTrqSC : Constant  Value=MWS.Shaft.PGB.TrqCoeff.CTrqSC
  CTrqSC1 : Constant  Value=MWS.Shaft.PGB.TrqCoeff.CTrqSC
  CTrqSR : Constant  Value=MWS.Shaft.PGB.TrqCoeff.CTrqSR
  CTrqSR1 : Constant  Value=MWS.Shaft.PGB.TrqCoeff.CTrqSR
  Compare To Constant : simulink/Logic and Bit Operations/Compare To Constant  relop=>=  const=5  OutDataTypeStr=boolean
  Compare To Zero : simulink/Logic and Bit Operations/Compare To Zero  relop=>=  OutDataTypeStr=boolean
  Constant{,34,36..37} (4 alike) : Constant  Value=MWS.In.Options.PGBConfig
  Constant1 : Constant  Value=[1 3]
  Constant{7..33} (27 alike) : Constant  Value=0
  Constant2 : Constant  Value=[1 2]
  Constant3 : Constant  Value=[2 3]
  Constant35 : Constant  Value=MWS.In.Options.EngineEMInt
  Constant4 : Constant  Value=[2 1]
  Constant5 : Constant  Value=[3 2]
  Constant6 : Constant  Value=[3 1]
  Data Type Conversion : DataTypeConversion  SaturateOnIntegerOverflow=off  RndMeth=Floor
  Demux : Demux  Outputs=2
  Demux1 : Demux
  Demux2 : Demux
  Demux3 : Demux  Outputs=2
  Demux4 : Demux  Outputs=2
  Divide{1,3,7..8,12..14} (7 alike) : Product  Inputs=*/
  Divide{2,4..6,9..10} (6 alike) : Product  Inputs=**/
  Gain{1..13} (13 alike) : Gain  Gain=-1
  Gearbox Speeds : Subsystem
  Memory : Memory  InitialCondition=[0 0]  InheritSampleTime=on
  Multiport Switch{,5..8} (5 alike) : MultiPortSwitch  Inputs=6  SaturateOnIntegerOverflow=off  InputSameDT=off
  Multiport Switch1 : MultiPortSwitch  SaturateOnIntegerOverflow=off  InputSameDT=off
  Multiport Switch2 : MultiPortSwitch  DataPortOrder=Specify indices  SaturateOnIntegerOverflow=off  InputSameDT=off
  Multiport Switch3 : MultiPortSwitch  DataPortOrder=Specify indices  SaturateOnIntegerOverflow=off  InputSameDT=off
  Multiport Switch4 : MultiPortSwitch  DataPortOrder=Specify indices  SaturateOnIntegerOverflow=off  InputSameDT=off
  Mux{,1..11} (12 alike) : Mux
  Mux{12..15} (4 alike) : Mux  Inputs=2
  Sign : Signum
  Spool Power Impact : Subsystem
  Sum : Sum  Inputs=|+-
  Sum1 : Sum  Inputs=|+-
  Sum2 : Sum  Inputs=|++
  Sum4 : Sum  Inputs=|+-
  Switch : Switch  Criteria=u2 > Threshold  SaturateOnIntegerOverflow=off  InputSameDT=off
  Switch1 : Switch  Criteria=u2 > Threshold  SaturateOnIntegerOverflow=off  InputSameDT=off
  Terminator : Terminator
  Terminator1 : Terminator
  While Iterator : WhileIterator  MaxIters=10  WhileBlockType=do-while  ShowIterationPort=on
  Zero2 : Constant
  PwrEPT_HP : Outport
  PwrEPT_LP : Outport  Port=2
  EPTsolver : Outport  Port=3
  wires:
  Constant/1 -> Multiport Switch/1
  Constant2/1 -> Multiport Switch/3
  Constant1/1 -> Multiport Switch/2
  Constant3/1 -> Multiport Switch/4
  Constant4/1 -> Multiport Switch/5
  Constant5/1 -> Multiport Switch/6
  Constant6/1 -> Multiport Switch/7
  Multiport Switch/1 -> Demux/1
  Demux/1 -> [HPID]  "HP component ID"
  Demux/2 -> [CoupID]  "Coupline component ID"
  CTrqSC/1 -> Divide3/1
  [NS] -> Divide13/2
  [NS] -> Divide7/2
  [NC] -> Divide8/2
  [NC] -> Divide3/2
  CTrqCR/1 -> Divide12/1
  [NR] -> Divide12/2
  [NR] -> Divide1/2
  CTrqCS/1 -> Divide13/1
  CTrqRS/1 -> Divide7/1
  CTrqRC/1 -> Divide8/1
  CTrqSR/1 -> Divide1/1
  Divide1/1 -> Multiport Switch2/3
  Divide3/1 -> Multiport Switch2/4
  Constant7/1 -> Multiport Switch2/2
  [CoupID] -> Multiport Switch2/1
  Divide7/1 -> Multiport Switch3/2
  Divide8/1 -> Multiport Switch3/4
  [CoupID] -> Multiport Switch3/1
  Constant8/1 -> Multiport Switch3/3
  Constant9/1 -> Multiport Switch4/4
  [CoupID] -> Multiport Switch4/1
  Divide13/1 -> Multiport Switch4/2
  Divide12/1 -> Multiport Switch4/3
  Multiport Switch3/1 -> Multiport Switch1/3
  Multiport Switch2/1 -> Multiport Switch1/2
  Multiport Switch4/1 -> Multiport Switch1/4
  [HPID] -> Multiport Switch1/1
  Multiport Switch1/1 -> Sign/1
  Sign/1 -> Compare To Zero/1
  Compare To Zero/1 -> [dirPwr]
  [dirPwr] -> Switch/2
  Gain1/1 -> Mux/2
  [PXpgb] -> Mux/1, Gain1/1
  Constant10/1 -> Mux/3
  Constant11/1 -> Mux/4
  Constant13/1 -> Mux1/4
  Constant12/1 -> Mux1/1
  [PXpgb] -> Mux1/2, Gain2/1
  Gain2/1 -> Mux1/3
  Constant14/1 -> Mux2/4
  [PXpgb] -> Mux2/3, Gain3/1
  Gain3/1 -> Mux2/2
  Constant15/1 -> Mux2/1
  [PXpgb] -> Mux3/1, Gain4/1
  Constant16/1 -> Mux3/4
  Gain4/1 -> Mux3/3
  Constant17/1 -> Mux3/2
  [PXpgb] -> Mux5/1, Gain6/1
  Constant19/1 -> Mux4/4
  [PXpgb] -> Mux4/2, Gain5/1
  Constant21/1 -> Mux5/4
  Gain6/1 -> Mux5/3
  Gain5/1 -> Mux4/1
  Constant20/1 -> Mux5/2
  Constant18/1 -> Mux4/3
  Constant24/1 -> Mux7/2
  Constant25/1 -> Mux7/4
  [PXpgb] -> Mux6/2, Gain7/1
  Constant23/1 -> Mux6/4
  [PXpgb] -> Mux7/3, Gain8/1
  Gain8/1 -> Mux7/1
  Gain7/1 -> Mux6/3
  Constant22/1 -> Mux6/1
  Gain9/1 -> Mux8/1
  Constant27/1 -> Mux8/4
  [PXpgb] -> Mux8/3, Gain9/1
  Gain10/1 -> Mux9/2
  Constant29/1 -> Mux9/4
  Constant26/1 -> Mux8/2
  [PXpgb] -> Gain10/1, Mux9/1
  Constant28/1 -> Mux9/3
  Constant32/1 -> Mux11/3
  [PXpgb] -> Mux11/2, Gain11/1
  Constant33/1 -> Mux11/4
  [PXpgb] -> Mux10/3, Gain12/1
  Constant31/1 -> Mux10/4
  Gain11/1 -> Mux11/1
  Gain12/1 -> Mux10/2
  Constant30/1 -> Mux10/1
  Mux1/1 -> [SRp]
  Mux/1 -> [SRn]
  Mux2/1 -> [SCp]
  Mux3/1 -> [SCn]
  Mux5/1 -> [RSp]
  Mux4/1 -> [RSn]
  Mux7/1 -> [RCp]
  Mux6/1 -> [RCn]
  Mux9/1 -> [CSp]
  Mux8/1 -> [CSn]
  Mux11/1 -> [CRp]
  Mux10/1 -> [CRn]
  [SCp] -> Multiport Switch6/2
  [SRp] -> Multiport Switch6/3
  [RCp] -> Multiport Switch6/4
  [RSp] -> Multiport Switch6/5
  [CRp] -> Multiport Switch6/6
  [CSp] -> Multiport Switch6/7
  [CSn] -> Multiport Switch7/7
  [CRn] -> Multiport Switch7/6
  [RSn] -> Multiport Switch7/5
  [RCn] -> Multiport Switch7/4
  [SRn] -> Multiport Switch7/3
  [SCn] -> Multiport Switch7/2
  Multiport Switch6/1 -> Switch/1
  Multiport Switch7/1 -> Switch/3
  Switch/1 -> Demux1/1
  Constant34/1 -> Multiport Switch7/1, Multiport Switch6/1
  Demux1/1 -> [PemS]
  Demux1/2 -> [PemR]
  Demux1/3 -> [PemC]
  Demux1/4 -> [PemP]
  [PemS] -> Spool Power Impact/1(PemS)
  [PemR] -> Spool Power Impact/2(PemR)
  [PemC] -> Spool Power Impact/3(PemC)
  [PemP] -> Spool Power Impact/4(PemP)
  [k_Alt] -> Gearbox Speeds/1(k_Alt)
  [f_Alt] -> Gearbox Speeds/2(f_Alt)
  [k_MN] -> Gearbox Speeds/3(k_MN)
  [f_MN] -> Gearbox Speeds/4(f_MN)
  [PwrBase_LP] -> Gearbox Speeds/5(PwrBase_LP)
  [PwrEPT_LPg] -> Gearbox Speeds/7(PwrEPT_LPg)
  [PwrBase_HP] -> Gearbox Speeds/6(PwrBase_HP)
  [PwrEPT_HPg] -> Gearbox Speeds/8(PwrEPT_HPg)
  Gearbox Speeds/1(NPGB) -> Demux2/1, [NPGB]
  Demux2/1 -> [NS]
  Demux2/3 -> [NC]
  Demux2/2 -> [NR]
  Demux2/4 -> Terminator/1
  [NPGB] -> Spool Power Impact/5(NPGB)
  k_Alt/1 -> [k_Alt]
  f_Alt/1 -> [f_Alt]
  k_MN/1 -> [k_MN]
  f_MN/1 -> [f_MN]
  PwrBase_LP/1 -> [PwrBase_LP]
  PwrBase_HP/1 -> [PwrBase_HP]
  [PwrEPT] -> Mux12/2, Gain13/1
  Switch1/1 -> Demux3/1
  Mux13/1 -> Switch1/1
  Mux12/1 -> Switch1/3
  Constant35/1 -> Switch1/2
  Demux3/2 -> PwrEPT_HP/1
  Demux3/1 -> PwrEPT_LP/1
  Spool Power Impact/1(PwrInLP) -> [PwrEPT_LP], Mux13/1
  Spool Power Impact/2(PwrInHP) -> Mux13/2, [PwrEPT_HP]
  PwrEPT/1 -> [PwrEPT]
  [PwrEPT_LPg] -> Sum/1
  [PwrEPT_LP] -> Sum/2
  [PwrEPT_HPg] -> Sum1/1
  [PwrEPT_HP] -> Sum1/2
  Sum/1 -> Abs/1
  Sum1/1 -> Abs1/1
  Abs/1 -> Sum2/1
  Abs1/1 -> Sum2/2
  Sum2/1 -> Mux15/1, [SumPwrErr]
  Memory/1 -> Demux4/1
  Demux4/1 -> [PwrEPT_LPg]
  Demux4/2 -> [PwrEPT_HPg]
  Mux14/1 -> Memory/1
  [PwrEPT_LP] -> Mux14/1
  [PwrEPT_HP] -> Mux14/2
  Compare To Constant/1 -> While Iterator/1
  [SumPwrErr] -> Compare To Constant/1
  While Iterator/1 -> Data Type Conversion/1
  Mux15/1 -> EPTsolver/1
  Data Type Conversion/1 -> Mux15/2
  Gain13/1 -> Mux12/1
  Zero2/1 -> Sum4/1
  CTrqSR1/1 -> Divide2/1
  [NC] -> Divide10/2
  [NR] -> Divide10/3
  Sum4/1 -> Divide14/2
  CTrqSC1/1 -> Divide4/1
  [NS] -> Divide2/2
  CTrqRS1/1 -> Divide5/1
  [NR] -> Divide5/2
  Divide5/1 -> [K_PXeffRS]
  [NS] -> Divide4/2
  Divide9/1 -> [K_PXeffCS]
  [PwrEPT] -> Divide14/1
  [K_PXeffSC] -> Multiport Switch5/2
  Multiport Switch5/1 -> [K_PXeffH]
  [K_PXeffSR] -> Multiport Switch5/3
  [NR] -> Divide6/2
  [K_PXeffRC] -> Multiport Switch5/4
  [K_PXeffCR] -> Multiport Switch5/6
  Constant36/1 -> Multiport Switch5/1
  CTrqCR1/1 -> Divide10/1
  [NS] -> Divide5/3
  CTrqRC1/1 -> Divide6/1
  [NC] -> Divide4/3
  Divide10/1 -> [K_PXeffCR]
  Divide2/1 -> [K_PXeffSR]
  [NR] -> Divide2/3
  [K_PXeffRS] -> Multiport Switch5/5
  [NS] -> Divide9/3
  [NC] -> Divide9/2
  CTrqCS1/1 -> Divide9/1
  [NC] -> Divide6/3
  [K_PXeffCS] -> Multiport Switch5/7
  Divide4/1 -> [K_PXeffSC]
  Divide6/1 -> [K_PXeffRC]
  Divide14/1 -> [PXpgb]
  [K_PXeffH] -> Sum4/2
  Constant37/1 -> Multiport Switch8/1
  [K_PXeffSR] -> Multiport Switch8/6
  [K_PXeffRC] -> Multiport Switch8/2
  [K_PXeffSC] -> Multiport Switch8/4
  Multiport Switch8/1 -> Terminator1/1
  [K_PXeffCR] -> Multiport Switch8/3
  [K_PXeffRS] -> Multiport Switch8/7
  [K_PXeffCS] -> Multiport Switch8/5

== system AGTF30SysDyn_PExPIn/Control System/Wf Controller/Controller/N1cSP Limit Controllers ==
  Prelookup : Inport
  N1 : Inport  Port=2
  N3 : Inport  Port=3
  Ps3 : Inport  Port=4
  T3 : Inport  Port=5
  T4 : Inport  Port=6
  T45 : Inport  Port=7
  N1cCmd : Inport  Port=8
  Mux : Mux  Inputs=7
  N1 Max Controller : Subsystem
  N3 Max Controller : Subsystem
  Ps3 Max Controller : Subsystem
  Ps3 Min Controller : Subsystem
  T3 Max Controller : Subsystem
  T4 Max Controller : Subsystem
  T45 Max Controller : Subsystem
  N1cSP T3 Max : Outport  VectorParamsAs1DForOutWhenUnconnected=off
  N1cSP T4 Max : Outport  Port=2  VectorParamsAs1DForOutWhenUnconnected=off
  N1cSP T45 Max : Outport  Port=3  VectorParamsAs1DForOutWhenUnconnected=off
  N1cSP N1 Max : Outport  Port=4  VectorParamsAs1DForOutWhenUnconnected=off
  N1cSP N3 Max : Outport  Port=5  VectorParamsAs1DForOutWhenUnconnected=off
  N1cSP Ps3 Max : Outport  Port=6  VectorParamsAs1DForOutWhenUnconnected=off
  N1cSP Ps3 Min : Outport  Port=7  VectorParamsAs1DForOutWhenUnconnected=off
  SPs : Outport  Port=8  VectorParamsAs1DForOutWhenUnconnected=off
  wires:
  T3 Max Controller/1(N1cDmd) -> N1cSP T3 Max/1
  T4 Max Controller/1(N1cDmd) -> N1cSP T4 Max/1
  Ps3 Min Controller/1(N1cDmd) -> N1cSP Ps3 Min/1
  N3 Max Controller/1(N1cDmd) -> N1cSP N3 Max/1
  Ps3 Max Controller/1(N1cDmd) -> N1cSP Ps3 Max/1
  T3 Max Controller/2(T3Max_SP) -> Mux/1  "T3Max"
  Mux/1 -> SPs/1
  N1 Max Controller/1(N1cDmd) -> N1cSP N1 Max/1
  N1/1 -> N1 Max Controller/2(N1)
  N3/1 -> N3 Max Controller/2(N3)
  T3/1 -> T3 Max Controller/2(T3)
  T4/1 -> T4 Max Controller/2(T4)
  Ps3/1 -> Ps3 Min Controller/2(Ps3), Ps3 Max Controller/2(Ps3)
  N1cCmd/1 -> T45 Max Controller/3(N1cCmd), Ps3 Min Controller/3(N1cCmd), Ps3 Max Controller/3(N1cCmd), N3 Max Controller/3(N1cCmd), N1 Max Controller/3(N1cCmd), T4 Max Controller/3(N1cCmd), T3 Max Controller/3(N1cCmd)
  T4 Max Controller/2(T4Max_SP) -> Mux/2  "T4Max"
  Ps3 Max Controller/2(Ps3Max_SP) -> Mux/6  "Ps3Max"
  N1 Max Controller/2(N1Max_SP) -> Mux/4  "N1Max"
  N3 Max Controller/2(N3Max_SP) -> Mux/5  "N3Max"
  Ps3 Min Controller/2(Ps3Min_SP) -> Mux/7  "Ps3Min"
  Prelookup/1 -> T45 Max Controller/1(Prelookup), Ps3 Min Controller/1(Prelookup), Ps3 Max Controller/1(Prelookup), N3 Max Controller/1(Prelookup), N1 Max Controller/1(Prelookup), T4 Max Controller/1(Prelookup), T3 Max Controller/1(Prelookup)
  T45/1 -> T45 Max Controller/2(T45)
  T45 Max Controller/2(T4Max_SP) -> Mux/3  "T45Max"
  T45 Max Controller/1(N1cDmd) -> N1cSP T45 Max/1

== system AGTF30SysDyn_PExPIn/Control System/Wf Controller/Controller/N1cSP Limit Select ==
  N1cSPReq : Inport
  Limits : Inport  Port=2
  Limit Selection : Lib_Cntrl_LimitSelect_TMATS/Limit Selection  SelectVec_M=MWS.Cntrl.WfCntrl.N1cSPLim.Type  LimitsEn_M=MWS.Cntrl.WfCntrl.N1cSPLim.En
  N1cSPdmd : Outport  VectorParamsAs1DForOutWhenUnconnected=off
  RegNum : Outport  Port=2  VectorParamsAs1DForOutWhenUnconnected=off
  wires:
  Limit Selection/2 -> RegNum/1
  Limit Selection/1 -> N1cSPdmd/1
  Limits/1 -> Limit Selection/2
  N1cSPReq/1 -> Limit Selection/1

== system AGTF30SysDyn_PExPIn/Control System/Wf Controller/Controller/Nominal Controller ==
  Prelookup : Inport
  N1cManEn : Inport  Port=2
  N1cMan : Inport  Port=3
  N1cSP : Inport  Port=4
  N1c : Inport  Port=5
  Wfcmd : Inport  Port=6
  Bus Selector : BusSelector  OutputSignals=k_PL,f_PL,k_Alt,f_Alt,k_MN,f_MN,k_PwrInLP,f_PwrInLP,k_PwrInHP,f_PwrInHP
  Constant : Constant  Value=MWS.Init.IC.Wf
  Discrete-Time Integrator : DiscreteIntegrator  SampleTime=MWS.In.Ts  ICPrevOutput=DiscIntNeverNeededParam  ICPrevScaledInput=DiscIntNeverNeededParam
  Divide2 : Product  Inputs=**
  Divide3 : Product  Inputs=**
  Gain : Gain  Gain=MWS.Cntrl.WfCntrl.Nom.Kiwp
  Ki Interpolation Using Prelookup : Interpolation_n-D  NumberOfTableDimensions=5  Table=MWS.Cntrl.WfCntrl.Nom.Ki_array  InternalRulePriority=Speed
      settings: InputPortMap=u0,u1,u2,u3,u4,u5,u6,u7,u8,u9
  Kp Interpolation Using Prelookup : Interpolation_n-D  NumberOfTableDimensions=5  Table=MWS.Cntrl.WfCntrl.Nom.Kp_array  InternalRulePriority=Speed
      settings: InputPortMap=u0,u1,u2,u3,u4,u5,u6,u7,u8,u9
  Sum : Sum  Inputs=|+-
  Sum1 : Sum  Inputs=|++
  Sum2 : Sum  Inputs=|-+
  Sum3 : Sum  Inputs=|+-
  Sum4 : Sum  Inputs=|++
  Switch : Switch  Criteria=u2 > Threshold  SaturateOnIntegerOverflow=off  InputSameDT=off
  Wfdmd : Outport  VectorParamsAs1DForOutWhenUnconnected=off
  N1cErr : Outport  Port=2  VectorParamsAs1DForOutWhenUnconnected=off
  wires:
  Ki Interpolation Using Prelookup/1 -> Divide2/1  "Ki"
  N1c/1 -> Sum/2
  Divide2/1 -> Discrete-Time Integrator/1
  Sum/1 -> N1cErr/1, [Error]
  Constant/1 -> Sum4/2
  Discrete-Time Integrator/1 -> Sum1/2
  Kp Interpolation Using Prelookup/1 -> Divide3/1  "Kp"
  Sum1/1 -> Sum4/1
  [Error] -> Divide3/2
  Divide3/1 -> Sum1/1
  Sum2/1 -> Gain/1
  Gain/1 -> Sum3/2
  Sum4/1 -> Sum2/2, Wfdmd/1
  [Error] -> Sum3/1
  Wfcmd/1 -> Sum2/1
  Sum3/1 -> Divide2/2
  Prelookup/1 -> Bus Selector/1
  Bus Selector/1 -> Ki Interpolation Using Prelookup/1, Kp Interpolation Using Prelookup/1  "<k_PL>"
  Bus Selector/2 -> Ki Interpolation Using Prelookup/2, Kp Interpolation Using Prelookup/2  "<f_PL>"
  Bus Selector/3 -> Ki Interpolation Using Prelookup/3, Kp Interpolation Using Prelookup/3  "<k_Alt>"
  Bus Selector/4 -> Ki Interpolation Using Prelookup/4, Kp Interpolation Using Prelookup/4  "<f_Alt>"
  Bus Selector/5 -> Ki Interpolation Using Prelookup/5, Kp Interpolation Using Prelookup/5  "<k_MN>"
  Bus Selector/6 -> Ki Interpolation Using Prelookup/6, Kp Interpolation Using Prelookup/6  "<f_MN>"
  Bus Selector/10 -> Ki Interpolation Using Prelookup/10, Kp Interpolation Using Prelookup/10  "<f_PwrInHP>"
  Bus Selector/7 -> Ki Interpolation Using Prelookup/7, Kp Interpolation Using Prelookup/7  "<k_PwrInLP>"
  Bus Selector/8 -> Ki Interpolation Using Prelookup/8, Kp Interpolation Using Prelookup/8  "<f_PwrInLP>"
  Bus Selector/9 -> Ki Interpolation Using Prelookup/9, Kp Interpolation Using Prelookup/9  "<k_PwrInHP>"
  Switch/1 -> Sum/1
  N1cSP/1 -> Switch/3  "N1cSP"
  N1cMan/1 -> Switch/1  "N1cSP"
  N1cManEn/1 -> Switch/2

== system AGTF30SysDyn_PExPIn/Control System/Wf Controller/Controller/Nominal Set-Point Determination ==
  Prelookup : Inport
  Bus Selector : BusSelector  OutputSignals=k_PL_Targ,f_PL_Targ,k_Alt,f_Alt,k_MN,f_MN,k_PwrInLP,f_PwrInLP,k_PwrInHP,f_PwrInHP
  NcFanSP Interpolation Using Prelookup : Interpolation_n-D  NumberOfTableDimensions=5  Table=MWS.Cntrl.WfCntrl.Sched.N1cSP.N1cSP_array  InternalRulePriority=Speed
      settings: InputPortMap=u0,u1,u2,u3,u4,u5,u6,u7,u8,u9
  N1cSP : Outport  VectorParamsAs1DForOutWhenUnconnected=off
  wires:
  Prelookup/1 -> Bus Selector/1
  Bus Selector/1 -> NcFanSP Interpolation Using Prelookup/1  "<k_PL_Targ>"
  Bus Selector/2 -> NcFanSP Interpolation Using Prelookup/2  "<f_PL_Targ>"
  Bus Selector/3 -> NcFanSP Interpolation Using Prelookup/3  "<k_Alt>"
  Bus Selector/4 -> NcFanSP Interpolation Using Prelookup/4  "<f_Alt>"
  Bus Selector/5 -> NcFanSP Interpolation Using Prelookup/5  "<k_MN>"
  Bus Selector/6 -> NcFanSP Interpolation Using Prelookup/6  "<f_MN>"
  Bus Selector/7 -> NcFanSP Interpolation Using Prelookup/7  "<k_PwrInLP>"
  Bus Selector/8 -> NcFanSP Interpolation Using Prelookup/8  "<f_PwrInLP>"
  Bus Selector/9 -> NcFanSP Interpolation Using Prelookup/9  "<k_PwrInHP>"
  Bus Selector/10 -> NcFanSP Interpolation Using Prelookup/10  "<f_PwrInHP>"
  NcFanSP Interpolation Using Prelookup/1 -> N1cSP/1
